simulink model "first_task"  (R2022a)
settings: Solver=VariableStepAuto  StartTime=0.0  StopTime=2.0  RelTol=1e-3
libraries: commsequence2 x1, commseqgen3 x1, dspspect3 x1, simulink x1, commutil2 x1
settings Model: Creator=Admin  LastModifiedBy=Admin

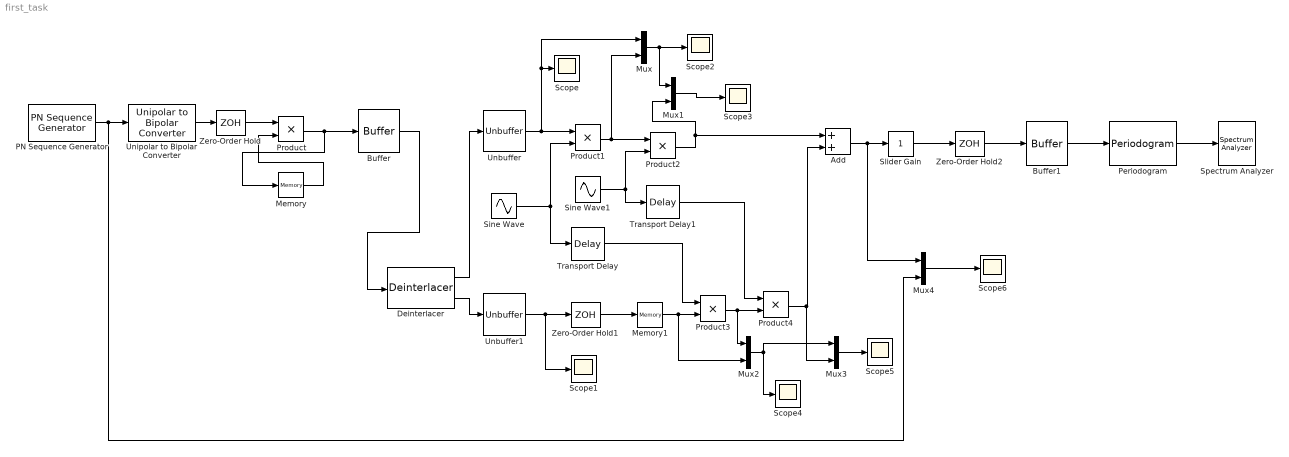
== system first_task ==
  Add : Sum
  Buffer : Buffer  N=2  OutputFrames=off
  Buffer1 : Buffer  N=2  OutputFrames=off
  Deinterlacer : commsequence2/Deinterlacer
      settings: SourceProductBaseCode=CM
  Memory : Memory  InitialCondition=1  InheritSampleTime=on
  Memory1 : Memory  InheritSampleTime=on
  Mux{,1..4} (5 alike) : Mux  Inputs=2
  PN Sequence Generator : commseqgen3/PN Sequence Generator  poly='z^6 + z + 1'  ini_sta=[0 0 0 0 0 1]  outBitMaskSource=Dialog parameter  shift=0  outVarSiz=off  maxOutSizeMode=Dialog parameter  maxOutSize=[10 1]  Ts=1/1200  sampPerFrame=1  reset=off  bitPackedOutputs=off  outDataType=double  numPackedBits=8  bitPackDataSigned=off  bitPackedOutDType=double
  Periodogram : dspspect3/Periodogram  measurement=Power spectral density  wintype=Hamming  Rs=50  beta=5  winsamp=Symmetric  FFTImplementation=Auto  inheritFFT=off  fftsize=256  navg=4  inheritTs=on  Ts=1
      settings: SourceProductBaseCode=DS
  Product{,1..4} (5 alike) : Product
  Scope{,1..6} (7 alike) : Scope
  Sine Wave : Sin  Frequency=600*pi  Phase=-pi  SampleTime=0
  Sine Wave1 : Sin  Frequency=76000*pi  SampleTime=0
  Slider Gain : simulink/Math Operations/Slider Gain  gain=1  low=0  high=2
  Spectrum Analyzer : SpectrumAnalyzer  IsFrequencyInputMode=1
  Transport Delay : TransportDelay  DelayTime=1/1200
  Transport Delay1 : TransportDelay  DelayTime=3/38000/4
  Unbuffer : Unbuffer
  Unbuffer1 : Unbuffer
  Unipolar to Bipolar Converter : commutil2/Unipolar to Bipolar Converter  M=2  polarity=Positive  dataType=Inherit via internal rule
  Zero-Order Hold : ZeroOrderHold  SampleTime=1/1200
  Zero-Order Hold1 : ZeroOrderHold  SampleTime=1/1200
  Zero-Order Hold2 : ZeroOrderHold  SampleTime=1/4000/3
  wires:
  PN Sequence Generator/1 -> Mux4/2, Unipolar to Bipolar Converter/1
  Unipolar to Bipolar Converter/1 -> Zero-Order Hold/1
  Zero-Order Hold/1 -> Product/1
  Product/1 -> Memory/1, Buffer/1
  Memory/1 -> Product/2
  Buffer/1 -> Deinterlacer/1
  Deinterlacer/1 -> Unbuffer/1
  Deinterlacer/2 -> Unbuffer1/1
  Unbuffer/1 -> Mux/1, Scope/1, Product1/1
  Sine Wave/1 -> Product1/2, Transport Delay/1
  Product1/1 -> Mux/2, Product2/1
  Unbuffer1/1 -> Scope1/1, Zero-Order Hold1/1
  Zero-Order Hold1/1 -> Memory1/1
  Memory1/1 -> Mux2/2, Product3/2
  Transport Delay/1 -> Product3/1
  Sine Wave1/1 -> Product2/2, Transport Delay1/1
  Product3/1 -> Mux2/1, Product4/2
  Transport Delay1/1 -> Product4/1
  Mux/1 -> Mux1/1, Scope2/1
  Mux1/1 -> Scope3/1
  Product2/1 -> Add/1, Mux1/2
  Product4/1 -> Mux3/2, Add/2
  Mux2/1 -> Scope4/1, Mux3/1
  Mux3/1 -> Scope5/1
  Add/1 -> Mux4/1, Slider Gain/1
  Slider Gain/1 -> Zero-Order Hold2/1
  Zero-Order Hold2/1 -> Buffer1/1
  Buffer1/1 -> Periodogram/1
  Mux4/1 -> Scope6/1
  Periodogram/1 -> Spectrum Analyzer/1
